simulink model "Modelo"  (R2025a)
settings: Solver=FixedStepAuto  StartTime=0.0  StopTime=10.0  FixedStep=.001  RelTol=1e-3
settings Model: Creator=aceve  LastModifiedBy=aceve

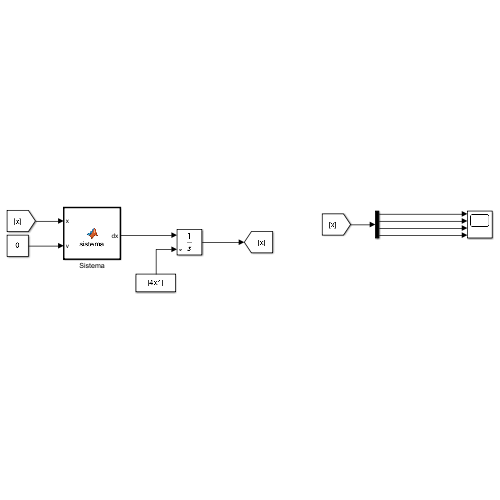
[thumbnail: Simulink's stored preview of the top-level diagram]
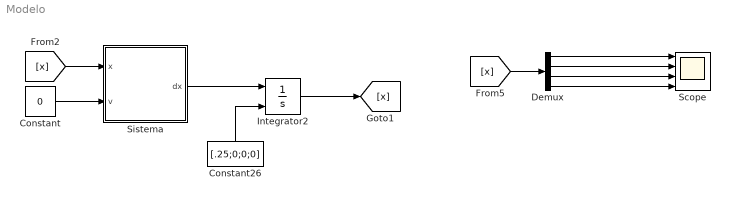
== system Modelo ==
  Constant : Constant  Value=0
  Constant26 : Constant  Value=[.25;0;0;0]
  Demux : Demux
  Integrator2 : Integrator  InitialConditionSource=external
  Scope : Scope  NumInputPorts=4
      settings: ActiveDisplayYMinimum=-16.783244283570824  ActiveDisplayYMaximum=16.783247205251637
  Sistema : MATLAB Function  TreatAsAtomicUnit=on
  wires:
  Constant26/1 -> Integrator2/2
  Sistema/1(dx) -> Integrator2/1
  Integrator2/1 -> [x]
  [x] -> Sistema/1(x)
  [x] -> Demux/1
  Demux/1 -> Scope/1
  Demux/2 -> Scope/2
  Constant/1 -> Sistema/2(v)
  Demux/3 -> Scope/3
  Demux/4 -> Scope/4

== matlab function Modelo/Sistema ==
  data: x input; dx output; v input
function dx = sistema(x, v)


dx = zeros(4,1);   % asegura tamaño fijo 4x1

M = 0.5;     % (M) Masa del carro (kg)
m = 0.2;     % (m) Masa del péndulo (kg)
l = 0.3;     % (l) Longitud del péndulo (m)
g = 9.81;    % (g) Gravedad (m/s^2)

th     = x(1);    % x1: ángulo péndulo
dth    = x(2);    % x2: velocidad angular péndulo
x_pos  = x(3);    % x3: posición carro
dx_pos = x(4);    % x4: velocidad carro


F_input = v(1);

s_th = sin(th);
c_th = cos(th);

% Denominador común
den_common = (m * s_th^2 + M);

% Calcular ddth (x2_dot)
num_x2 = F_input*c_th + (M+m)*g*s_th - m*l*dth^2*s_th*c_th;
den_x2 = den_common * l;
ddth = num_x2 / den_x2;

% Calcular ddx_pos (x4_dot)
num_x4 = F_input + m*g*s_th*c_th - m*l*dth^2*s_th;
den_x4 = den_common;
ddx_pos = num_x4 / den_x4;

%% ---- Derivadas de estado ----
dx(1) = dth;
dx(2) = ddth;
dx(3) = dx_pos;
dx(4) = ddx_pos;

end
